simulink model "l4"  (R2013a)
settings: Solver=ode45  StartTime=0.0  StopTime=30  RelTol=1e-3
settings Model: Creator=Sion  LastModifiedBy=Sion

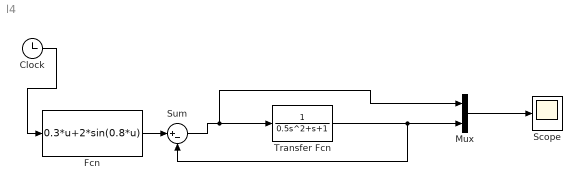
== system l4 ==
  Clock : Clock
  Fcn : Fcn  Expr=0.3*u+2*sin(0.8*u)
  Mux : Mux  Inputs=2
  Scope : Scope
      settings: TimeRange=30  YMin=-2.41672e-62  YMax=10  SaveName=ScopeData25
  Sum : Sum  Inputs=|+-
  Transfer Fcn : TransferFcn  Denominator=[0.5 1 1]
  wires:
  Transfer Fcn/1 -> Mux/2, Sum/2
  Fcn/1 -> Sum/1
  Sum/1 -> Mux/1, Transfer Fcn/1
  Clock/1 -> Fcn/1
  Mux/1 -> Scope/1
